simulink model "motor_control_position"  (R2019b)
settings: Solver=VariableStepAuto  StartTime=0.0  StopTime=1.0  RelTol=1e-3
undefined symbols (not defined in the file): Bnew, Gear_Ratio, Jnew, Kd_position, Ke, Ki_current, Ki_velocity, Kp_current, Kp_position, Kp_velocity, Kt, La, Ra, V
libraries: simulink_extras x4
settings Model: Creator=이종수  LastModifiedBy=이종수

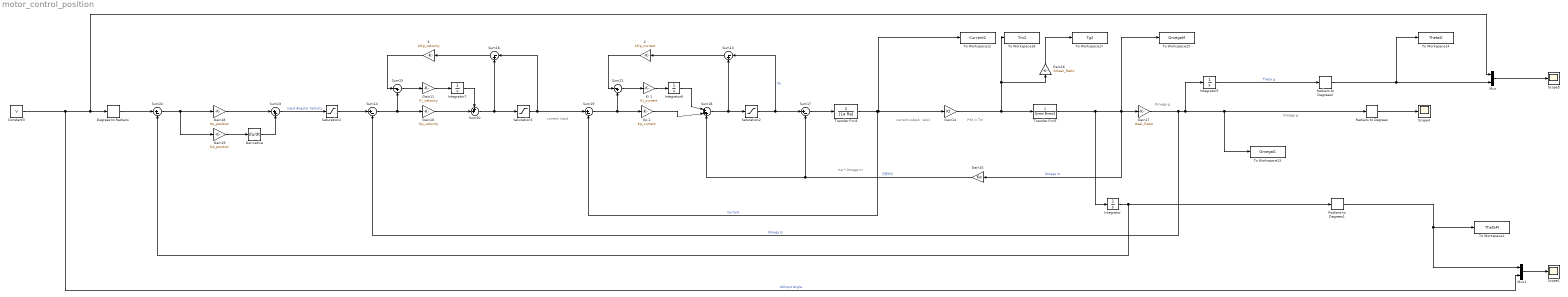
== system motor_control_position ==
  note: current output : Ia(s)
  note: I*Kt = Tm
  note: Omega g
  note: Ke * Omega m
  note: Omega g
  note: current input
  " 2" : Gain  Gain=1/Kp_current
  " 3" : Gain  Gain=1/Kp_velocity
  Constant3 : Constant  Value=V
  Degrees to Radians : simulink_extras/Transformations/Degrees to Radians
  Derivative : Derivative
  Gain10 : Gain  Gain=Kp_velocity
  Gain11 : Gain  Gain=Ki_velocity
  Gain14 : Gain  Gain=Kt
  Gain15 : Gain  Gain=Ke
  Gain16 : Gain  Gain=1/Gear_Ratio
  Gain17 : Gain  Gain=Gear_Ratio
  Gain18 : Gain  Gain=Kp_position
  Gain19 : Gain  Gain=Kd_position
  Integrator{,5..7} (4 alike) : Integrator
  Ki 1 : Gain  Gain=Ki_current
  Kp 1 : Gain  Gain=Kp_current
  Mux : Mux  Inputs=2
  Mux1 : Mux  Inputs=2
  Radians to Degrees : simulink_extras/Transformations/Radians to Degrees
  Radians to Degrees1 : simulink_extras/Transformations/Radians to Degrees
  Radians to Degrees2 : simulink_extras/Transformations/Radians to Degrees
  Saturation1 : Saturate  UpperLimit=642.98  LowerLimit=-642.98
  Saturation2 : Saturate  UpperLimit=48  LowerLimit=-48
  Saturation3 : Saturate  UpperLimit=27.3  LowerLimit=-27.3
  Scope1 : Scope
  Scope4 : Scope
  Scope5 : Scope
  Sum{13,15..16,21} (4 alike) : Sum  Inputs=|-+
  Sum{14,17,19,22} (4 alike) : Sum  Inputs=|+-
  Sum18 : Sum  Inputs=|+++
  Sum20 : Sum  Inputs=++|
  Sum23 : Sum  Inputs=|++
  To Workspace1 : ToWorkspace  VariableName=ThetaM  SaveFormat=Structure With Time  SampleTime=-1
  To Workspace12 : ToWorkspace  VariableName=Current2  SaveFormat=Structure With Time  SampleTime=-1
  To Workspace13 : ToWorkspace  VariableName=OmegaG  SaveFormat=Structure With Time  SampleTime=-1
  To Workspace14 : ToWorkspace  VariableName=ThetaG  SaveFormat=Structure With Time  SampleTime=-1
  To Workspace15 : ToWorkspace  VariableName=OmegaM  SaveFormat=Structure With Time  SampleTime=-1
  To Workspace16 : ToWorkspace  VariableName=Tm2  SaveFormat=Structure With Time  SampleTime=-1
  To Workspace17 : ToWorkspace  VariableName=Tg2  SaveFormat=Structure With Time  SampleTime=-1
  Transfer Fcn4 : TransferFcn  Denominator=[La Ra]
  Transfer Fcn5 : TransferFcn  Denominator=[Jnew Bnew]
  wires:
  Integrator6/1 -> Sum18/1
  Gain16/1 -> To Workspace17/1
  Sum23/1 -> Saturation1/1  "Input Angular Velocity"
  Transfer Fcn5/1 -> To Workspace15/1, Gain15/1, Gain17/1, Integrator/1  "Omega m"
  Sum14/1 -> Sum15/2, Gain10/1
  Sum20/1 -> Sum16/2, Saturation3/1
  Sum19/1 -> Kp 1/1, Sum21/2
  Ki 1/1 -> Integrator6/1
  Sum18/1 -> Sum13/2, Saturation2/1
  Transfer Fcn4/1 -> Gain14/1, To Workspace12/1, Sum19/2  "Current"
  Gain14/1 -> Transfer Fcn5/1, Gain16/1, To Workspace16/1
  Gain15/1 -> Sum18/3, Sum17/2  "전향보상"
  Integrator5/1 -> Radians to Degrees2/1  "Theta g"
  Saturation2/1 -> Sum13/1, Sum17/1  "Va"
  Sum17/1 -> Transfer Fcn4/1
  " 2"/1 -> Sum21/1
  Gain11/1 -> Integrator7/1
  Integrator7/1 -> Sum20/1
  " 3"/1 -> Sum15/1
  Kp 1/1 -> Sum18/2
  Gain10/1 -> Sum20/2
  Gain17/1 -> To Workspace13/1, Radians to Degrees/1, Integrator5/1, Sum14/2  "Omega G"
  Saturation3/1 -> Sum16/1, Sum19/1
  Sum13/1 -> " 2"/1
  Sum15/1 -> Gain11/1
  Sum16/1 -> " 3"/1
  Sum21/1 -> Ki 1/1
  Constant3/1 -> Mux1/2, Degrees to Radians/1, Mux/1  "ddInput Angle"
  Gain19/1 -> Derivative/1
  Gain18/1 -> Sum23/1
  Derivative/1 -> Sum23/2
  Sum22/1 -> Gain19/1, Gain18/1
  Mux/1 -> Scope5/1
  Degrees to Radians/1 -> Sum22/1
  Radians to Degrees/1 -> Scope4/1
  Mux1/1 -> Scope1/1
  Saturation1/1 -> Sum14/1
  Integrator/1 -> Radians to Degrees1/1, Sum22/2
  Radians to Degrees1/1 -> Mux1/1, To Workspace1/1
  Radians to Degrees2/1 -> To Workspace14/1, Mux/2
